simulink model "Kalman_Artefact_Simple"  (R2019b)
settings: Solver=VariableStepAuto  StartTime=0.0  StopTime=4  FixedStep=0.01  RelTol=1e-3
values from neighbouring files (symbols this model uses):
  A = [Ae zeros(p, ro); zeros(ro, p) At]    [Kalman.m]    (also in Kalman_EMG.m; Kalman_Phase.m = a*eye(2*num_rhythms)*O)
  B = [zeros(p, 1); Bt]    [Kalman.m]    (also in Kalman_EMG.m; Kalman_Phase.m = zeros(2*num_rhythms))
  C = [Ce Ct]    [Kalman.m]    (also in Kalman_EMG.m; Kalman_Phase.m = M)
  end_samples = 30000    [Kalman_EMG.m]
  Gm = [Ge zeros(p, ro); zeros(ro, 1) eye(ro)]    [Kalman.m]    (also in Kalman_EMG.m; Kalman_Phase.m = Q)
  Ts = y_arm.interval    [Kalman.m]    (also in Kalman_EMG.m; Kalman_Phase.m = 0.0001)
libraries: dspsrcs4 x8
settings Model: Creator=isidoraradenkovic  LastModifiedBy=isidoraradenkovic
settings DataIOCC: ReturnWorkspaceOutputs=off
settings OptimizationCC: DefaultParameterBehavior=Inlined  PassReuseOutputArgsAs=Individual arguments  EfficientTunableParamExpr=on
settings DebuggingCC: ParameterTunabilityLossMsg=error  ArithmeticOperatorsInVariantConditions=warning
settings SFSimCC: SimUseLocalCustomCode=off  MATLABDynamicMemAlloc=off  CustomCodeUndefinedFunction=UseInterfaceOnly
settings RTWCC: SystemTargetFile=ert.tlc  TemplateMakefile=ert_default_tmf  GenerateReport=on  RTWUseLocalCustomCode=off  IncludeHyperlinkInReport=on  LaunchReport=on  GenerateTraceInfo=on  GenerateTraceReport=on  GenerateTraceReportSl=on  GenerateTraceReportSf=on  GenerateTraceReportEml=on  CheckMdlBeforeBuild=Warning
settings CodeAppCC: GenerateComments=off  IgnoreCustomStorageClasses=off  SimulinkBlockComments=off
settings ERTTargetCC: TargetLangStandard=C99 (ISO)  GenerateSampleERTMain=on  InlinedParameterPlacement=NonHierarchical  ERTCustomFileTemplate=example_file_process.tlc
settings SimscapeCC: SimscapeNormalizeSystem=off

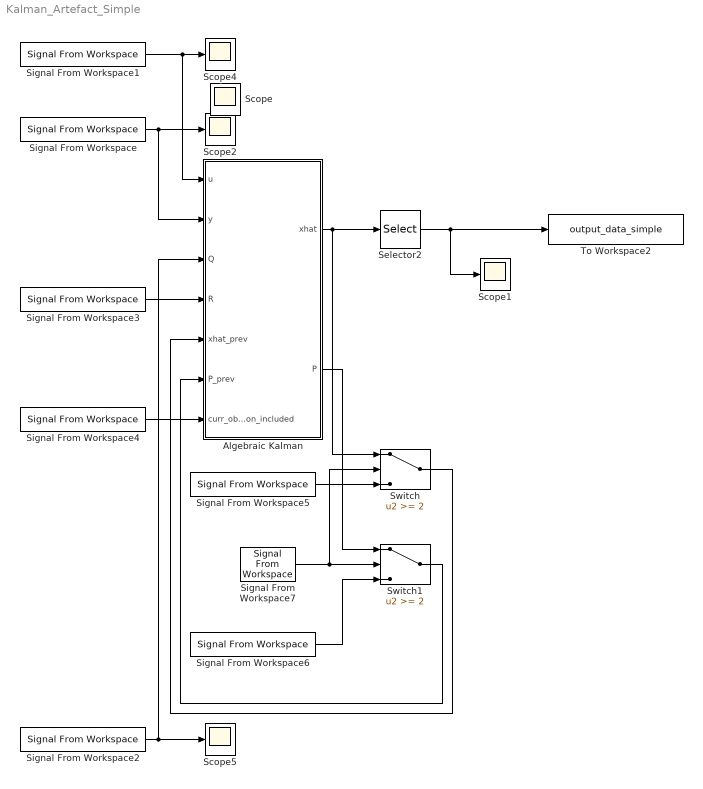
== system Kalman_Artefact_Simple ==
  Algebraic Kalman : MATLAB Function  TreatAsAtomicUnit=on
  Scope{,1..2,4..5} (5 alike) : Scope
  Selector2 : Selector  InputPortWidth=6  IndexOptions=Index vector (dialog)  Indices=[1]  OutputSizes=1
  Signal From Workspace : dspsrcs4/Signal From Workspace  X=input_data  Ts=Ts  nsamps=1  OutputAfterFinalValue=Cyclic repetition  ignoreOrWarnInputAndFrameLengths=off  OutputFrames=off
  Signal From Workspace1 : dspsrcs4/Signal From Workspace  X=tms_pulses  Ts=Ts  nsamps=1  OutputAfterFinalValue=Cyclic repetition  ignoreOrWarnInputAndFrameLengths=off  OutputFrames=off
  Signal From Workspace2 : dspsrcs4/Signal From Workspace  X=Q  Ts=Ts/4  nsamps=4  OutputAfterFinalValue=Cyclic repetition  ignoreOrWarnInputAndFrameLengths=off  OutputFrames=off
  Signal From Workspace3 : dspsrcs4/Signal From Workspace  X=R  Ts=Ts  nsamps=1  OutputAfterFinalValue=Cyclic repetition  ignoreOrWarnInputAndFrameLengths=off  OutputFrames=off
  Signal From Workspace4 : dspsrcs4/Signal From Workspace  X=1  Ts=Ts  nsamps=1  OutputAfterFinalValue=Cyclic repetition  ignoreOrWarnInputAndFrameLengths=off  OutputFrames=off
  Signal From Workspace5 : dspsrcs4/Signal From Workspace  X=x0  Ts=Ts  nsamps=1  OutputAfterFinalValue=Cyclic repetition  ignoreOrWarnInputAndFrameLengths=off  OutputFrames=off
  Signal From Workspace6 : dspsrcs4/Signal From Workspace  X=P0  Ts=Ts/6  nsamps=6  OutputAfterFinalValue=Cyclic repetition  ignoreOrWarnInputAndFrameLengths=off  OutputFrames=off
  Signal From Workspace7 : dspsrcs4/Signal From Workspace  X=1:1:end_samples  Ts=Ts  nsamps=1  OutputAfterFinalValue=Cyclic repetition  ignoreOrWarnInputAndFrameLengths=off  OutputFrames=off
  Switch : Switch  Threshold=2
  Switch1 : Switch  Threshold=2
  To Workspace2 : ToWorkspace  VariableName=output_data_simple  SampleTime=-1
      settings: Save2DSignal=2-D array (concatenate along first dimension)
  wires:
  Signal From Workspace2/1 -> Scope5/1, Algebraic Kalman/3(Q)
  Signal From Workspace3/1 -> Algebraic Kalman/4(R)
  Signal From Workspace1/1 -> Algebraic Kalman/1(u), Scope4/1
  Algebraic Kalman/1(xhat) -> Selector2/1, Switch/1
  Selector2/1 -> Scope1/1, To Workspace2/1
  Signal From Workspace7/1 -> Switch/2, Switch1/2
  Signal From Workspace4/1 -> Algebraic Kalman/7(curr_observation_included)
  Signal From Workspace/1 -> Scope2/1, Algebraic Kalman/2(y)
  Switch1/1 -> Algebraic Kalman/6(P_prev)
  Switch/1 -> Algebraic Kalman/5(xhat_prev)
  Algebraic Kalman/2(P) -> Switch1/1
  Signal From Workspace5/1 -> Switch/3
  Signal From Workspace6/1 -> Switch1/3

== matlab function Kalman_Artefact_Simple/Algebraic Kalman ==
  data: u input; xhat output; y input; Q input; R input; xhat_prev input; P_prev input; curr_observation_included input; P output; A parameter; B parameter; C parameter; Gm parameter
function [xhat, P] = algebraic_kalman(u, y, Q, R, xhat_prev, P_prev, curr_observation_included, A, B, C, Gm)
x_time = A*xhat_prev + B*u;
P_time = A*P_prev*A'+ Gm*Q*Gm';

K = P_time*(C')*pinv(C*P_time*C' + R);
epsilon = y - C*x_time;

if curr_observation_included
    xhat = x_time + K*epsilon;
    P = P_time - K*C*P_time;
else
    xhat = x_time;
    P = P_time;
end
